simulink model "simplified_model"  (R2018b)
settings: Solver=VariableStepAuto  StartTime=0.0  StopTime=20  RelTol=1e-3
settings Model: Creator=dylan  LastModifiedBy=dylan

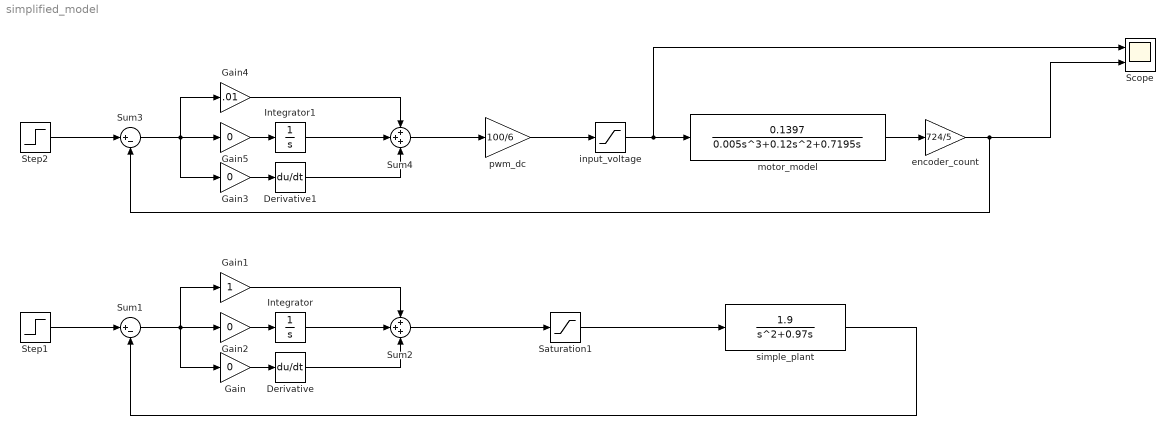
== system simplified_model ==
  Derivative : Derivative
  Derivative1 : Derivative
  Gain{,2..3,5} (4 alike) : Gain  Gain=0
  Gain1 : Gain
  Gain4 : Gain  Gain=.01
  Integrator : Integrator
  Integrator1 : Integrator
  Saturation1 : Saturate  UpperLimit=6  LowerLimit=-6
  Scope : Scope  NumInputPorts=2
  Step1 : Step  SampleTime=0
  Step2 : Step  After=2*pi*724/5  SampleTime=0
  Sum1 : Sum  Inputs=|+-
  Sum2 : Sum  Inputs=+++
  Sum3 : Sum  Inputs=|+-
  Sum4 : Sum  Inputs=+++
  encoder_count : Gain  Gain=724/5
  input_voltage : Saturate  UpperLimit=6  LowerLimit=-6
  motor_model : TransferFcn  Numerator=[0.1397]  Denominator=[0.005 0.12 0.7195 0]
  pwm_dc : Gain  Gain=100/6
  simple_plant : TransferFcn  Numerator=[1.9]  Denominator=[1 0.97 0]
  wires:
  Step1/1 -> Sum1/1
  simple_plant/1 -> Sum1/2
  Gain/1 -> Derivative/1
  Gain2/1 -> Integrator/1
  Gain1/1 -> Sum2/1
  Integrator/1 -> Sum2/2
  Derivative/1 -> Sum2/3
  Sum1/1 -> Gain/1, Gain2/1, Gain1/1
  Integrator1/1 -> Sum4/2
  Gain4/1 -> Sum4/1
  Sum3/1 -> Gain3/1, Gain5/1, Gain4/1
  Gain5/1 -> Integrator1/1
  Derivative1/1 -> Sum4/3
  Step2/1 -> Sum3/1
  Gain3/1 -> Derivative1/1
  input_voltage/1 -> Scope/1, motor_model/1
  Saturation1/1 -> simple_plant/1
  Sum2/1 -> Saturation1/1
  motor_model/1 -> encoder_count/1
  encoder_count/1 -> Scope/2, Sum3/2
  pwm_dc/1 -> input_voltage/1
  Sum4/1 -> pwm_dc/1
